simulink model "generate_model"  (R2015b)
settings: Solver=FixedStepAuto  StartTime=0.0  StopTime=10.0  RelTol=1e-3
undefined symbols (not defined in the file or in its folder): A_sine, A_step, A_triangle, A_variant, const_variant, den, f_sine, k_noise, k_ramp, k_sine, k_step, k_triangle, k_variant, num, slope_ramp, Ts
libraries: simulink x2, powerlib_meascontrol x1
settings Model: Creator=start  LastModifiedBy=start

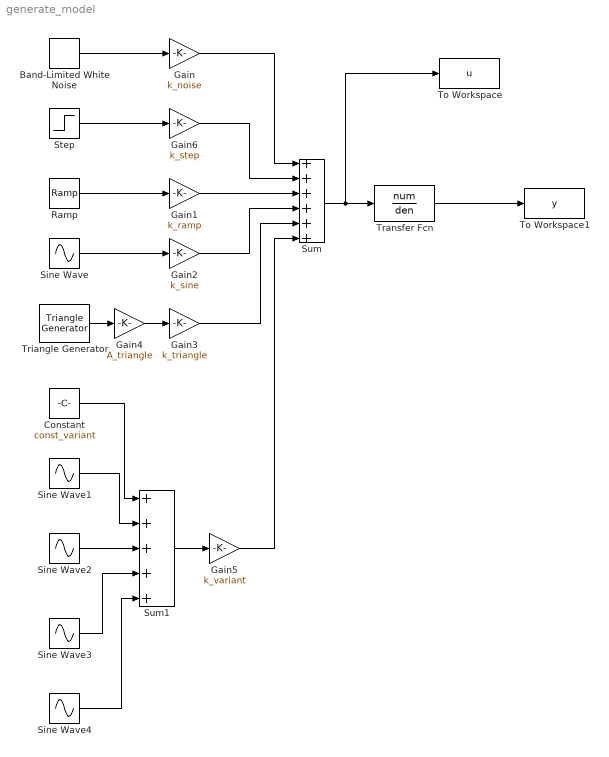
== system generate_model ==
  Band-Limited White Noise : simulink/Sources/Band-Limited White Noise  Cov=A_noise  Ts=Ts  seed=[23341]
  Constant : Constant  Value=const_variant
  Gain : Gain  Gain=k_noise
  Gain1 : Gain  Gain=k_ramp
  Gain2 : Gain  Gain=k_sine
  Gain3 : Gain  Gain=k_triangle
  Gain4 : Gain  Gain=A_triangle
  Gain5 : Gain  Gain=k_variant
  Gain6 : Gain  Gain=k_step
  Ramp : simulink/Sources/Ramp  slope=slope_ramp  start=0  X0=0.1
  Sine Wave : Sin  Amplitude=A_sine  Frequency=f_sine  Phase=pi/2  SampleTime=Ts
  Sine Wave1 : Sin  Amplitude=0.5*A_variant  SampleTime=0
  Sine Wave2 : Sin  Amplitude=0.2*A_variant  Frequency=2.5  SampleTime=0
  Sine Wave3 : Sin  Amplitude=0.25*A_variant  Frequency=0.2  SampleTime=0
  Sine Wave4 : Sin  Amplitude=0.05*A_variant  Frequency=2  SampleTime=0
  Step : Step  Time=0  After=A_step  SampleTime=0
  Sum : Sum  Inputs=++++++
  Sum1 : Sum  Inputs=+++++
  To Workspace : ToWorkspace  VariableName=u  SaveFormat=Structure With Time  SampleTime=-1
  To Workspace1 : ToWorkspace  VariableName=y  SaveFormat=Structure With Time  SampleTime=-1
  Transfer Fcn : TransferFcn  Numerator=num  Denominator=den
  Triangle Generator : powerlib_meascontrol/Pulse & Signal Generators/Triangle Generator  Freq=f_triangle  Phase=180  Ts=Ts
  wires:
  Ramp/1 -> Gain1/1
  Sine Wave/1 -> Gain2/1
  Triangle Generator/1 -> Gain4/1
  Sum/1 -> To Workspace/1, Transfer Fcn/1
  Transfer Fcn/1 -> To Workspace1/1
  Band-Limited White Noise/1 -> Gain/1
  Gain4/1 -> Gain3/1
  Constant/1 -> Sum1/1
  Sine Wave1/1 -> Sum1/2
  Sine Wave2/1 -> Sum1/3
  Sine Wave3/1 -> Sum1/4
  Sine Wave4/1 -> Sum1/5
  Sum1/1 -> Gain5/1
  Step/1 -> Gain6/1
  Gain1/1 -> Sum/3
  Gain2/1 -> Sum/4
  Gain6/1 -> Sum/2
  Gain3/1 -> Sum/5
  Gain/1 -> Sum/1
  Gain5/1 -> Sum/6
